simulink model "flyback_switching"  (R2019b)
settings: Solver=FixedStepDiscrete  StartTime=0.0  StopTime=1/60  FixedStep=Ts/1000  MaxStep=1e-4  RelTol=1e-3
values from neighbouring files (symbols this model uses):
  n1 = 2    [final_params.m]
  np = 7    [final_params.m]
  Ts = 1/fsw    (= 1e-05)    [final_params.m]
undefined symbols (not defined in the file or in its folder): C, Cf, duty, fL, Lf, Lm, Vgrms
libraries: powerlib x19, powerlib_meascontrol x1
settings Model: Creator=jvr2131  LastModifiedBy=john
settings DataIOCC: ReturnWorkspaceOutputs=off
settings DebuggingCC: ArithmeticOperatorsInVariantConditions=warning
settings SFSimCC: SimUseLocalCustomCode=off  CustomCodeUndefinedFunction=UseInterfaceOnly
settings RTWCC: RTWUseLocalCustomCode=off

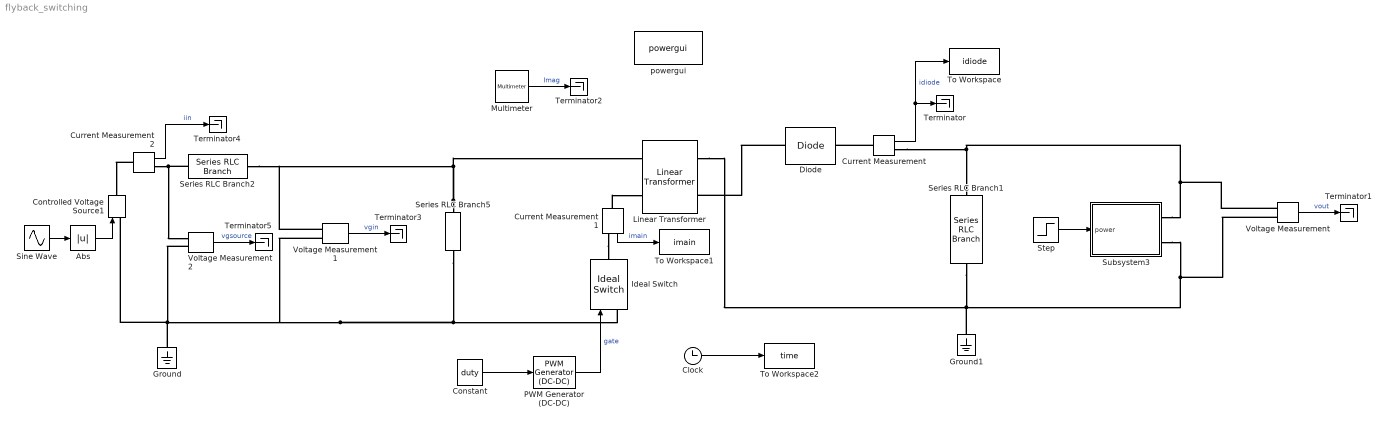
== system flyback_switching ==
  Abs : Abs
  Clock : Clock
  Constant : Constant  Value=duty
  Controlled Voltage Source1 : powerlib/Electrical Sources/Controlled Voltage Source  Initialize=on  Source_Type=AC  Amplitude=0  Phase=0  Frequency=0  Measurements=None
      settings: SourceProductName=Simscape Electrical
  Current Measurement : powerlib/Measurements/Current Measurement  PhasorSimulation=off  OutputType=Complex  PSBequivalent=0
      settings: SourceProductName=Simscape Electrical
  Current Measurement1 : powerlib/Measurements/Current Measurement  PhasorSimulation=off  OutputType=Complex  PSBequivalent=0
      settings: SourceProductName=Simscape Electrical
  Current Measurement2 : powerlib/Measurements/Current Measurement  PhasorSimulation=off  OutputType=Complex  PSBequivalent=0
      settings: SourceProductName=Simscape Electrical
  Diode : powerlib/Power Electronics/Diode  Ron=0.001  Lon=0  Vf=0  IC=0  UseSnubber=0  Rs=500  Cs=0  Measurements=off
      settings: SourceProductName=Simscape Electrical
  Ground : powerlib/Elements/Ground  LConnTagsString=a
      settings: SourceProductName=Simscape Electrical
  Ground1 : powerlib/Elements/Ground  LConnTagsString=a
      settings: SourceProductName=Simscape Electrical
  Ideal Switch : powerlib/Power Electronics/Ideal Switch  Ron=0.001  Lon=0  IC=0  Rs=1e5  Cs=inf  Measurements=off
      settings: SourceProductName=Simscape Electrical
  Linear Transformer : powerlib/Elements/Linear Transformer  UNITS=SI  NominalPower=[ 250e6 60 ]  winding1=[7.35e+05 0 0]  winding2=[(n1/np)*7.35e+05 0 0]  ThreeWindings=off  winding3=[3.15e+05 0.7938 0.084225]  RmLm=[1.0805e+06 Lm]  Measurements=Magnetization current  DataType=on
      settings: SourceProductName=Simscape Electrical
  Multimeter : powerlib/Measurements/Multimeter  PhasorSimulation=off  OutputType=Complex  sel=2  L=3  Gain=1  yselected={'Imag: Linear Transformer'};  PSBOutputType=1  PSBequivalent=0  AxesSetting=[0,0.1,-100,100]  Display=0  SavedBlockNames=-11
      settings: SourceProductName=Simscape Electrical
  PWM Generator (DC-DC) : powerlib_meascontrol/Pulse & Signal Generators/PWM Generator (DC-DC)  Fsw=fs  Ts=0
      settings: SourceProductName=Simscape Electrical
  Series RLC Branch1 : powerlib/Elements/Series RLC Branch  LConnTagsString=__new0  RConnTagsString=__new0  BranchType=C  Resistance=1  Inductance=1e-3  SetiL0=off  InitialCurrent=0  Capacitance=0.1  Setx0=on  InitialVoltage=V  Measurements=None
      settings: SourceProductName=Simscape Electrical
  Series RLC Branch2 : powerlib/Elements/Series RLC Branch  LConnTagsString=__new0  RConnTagsString=__new0  BranchType=L  Resistance=1  Inductance=Lf  SetiL0=off  InitialCurrent=0  Capacitance=C  Setx0=on  InitialVoltage=V  Measurements=None
      settings: SourceProductName=Simscape Electrical
  Series RLC Branch5 : powerlib/Elements/Series RLC Branch  LConnTagsString=__new0  RConnTagsString=__new0  BranchType=C  Resistance=1  Inductance=1e-3  SetiL0=off  InitialCurrent=0  Capacitance=Cf  Setx0=off  InitialVoltage=V  Measurements=None
      settings: SourceProductName=Simscape Electrical
  Sine Wave : Sin  Amplitude=Vgrms*sqrt(2)  Frequency=2*pi*fL  SampleTime=0
  Step : Step  Time=0  Before=power  After=power  SampleTime=0
  Subsystem3 : Subsystem
  Terminator{,1..5} (6 alike) : Terminator
  To Workspace : ToWorkspace  VariableName=idiode  SampleTime=-1
  To Workspace1 : ToWorkspace  VariableName=imain  SampleTime=-1
  To Workspace2 : ToWorkspace  VariableName=time  SampleTime=-1
  Voltage Measurement : powerlib/Measurements/Voltage Measurement  PhasorSimulation=off  OutputType=Complex  PSBequivalent=0
      settings: SourceProductName=Simscape Electrical
  Voltage Measurement1 : powerlib/Measurements/Voltage Measurement  PhasorSimulation=off  OutputType=Complex  PSBequivalent=0
      settings: SourceProductName=Simscape Electrical
  Voltage Measurement2 : powerlib/Measurements/Voltage Measurement  PhasorSimulation=off  OutputType=Complex  PSBequivalent=0
      settings: SourceProductName=Simscape Electrical
  powergui : powerlib/powergui  Priority=1  SimulationMode=Discrete  SampleTime=Ts/1000  frequency=60  Iterations=50  frequencyindice=0  Pbase=100e6  ErrMax=1e-4  UnitsV=kV  UnitsW=MW  buscounter=0  FunctionMessages=off  echomessages=off  EnableUseOfTLC=off  CurrentSourceSwitches=off  DisableSnubberDevices=off  DisableRonSwitches=off  DisableVfSwitches=off  DisplayEquations=off  AutomaticDiscreteSolvers=off  SolverType=Tustin/Backward Euler (TBE)  Interpol=off  ExternalGateDelay=off  methode=off  Ts=100  x0status=blocks  SPID=on  SwTol=0  HookPort=off  NonlinearTolerance=1e-4  nMaxIteration=100  ContinueOnMaxIteration=off  RestoreLinks=warning  ResistiveCurrentMeasurement=off  Frange=[0:2:500]  Ylog=off  Xlog=on  ShowGrid=off  save=off  variable=ZData  structure=0  ZoomFFT=off  StartTime=0.0  cycles=1  DisplayStyle=1  fundamental=60  FreqAxis=off  MaxFrequency=1000  frequencyindicesteady=1  RmsSteady=1  display=off
      settings: SourceProductName=Simscape Electrical
  wires:
  Current Measurement/1 -> To Workspace/1, Terminator/1  "idiode"
  Voltage Measurement/1 -> Terminator1/1  "vout"
  PWM Generator (DC-DC)/1 -> Ideal Switch/1  "gate"
  Constant/1 -> PWM Generator (DC-DC)/1
  Multimeter/1 -> Terminator2/1  "Imag"
  Step/1 -> Subsystem3/1(power)
  Voltage Measurement1/1 -> Terminator3/1  "vgin"
  Current Measurement1/1 -> To Workspace1/1  "imain"
  Sine Wave/1 -> Abs/1
  Abs/1 -> Controlled Voltage Source1/1
  Clock/1 -> To Workspace2/1
  Current Measurement2/1 -> Terminator4/1  "iin"
  Voltage Measurement2/1 -> Terminator5/1  "vgsource"
  connections:
  Series RLC Branch5/RConn1 -- Ideal Switch/LConn1 -- Voltage Measurement2/LConn2 -- Controlled Voltage Source1/LConn1 -- Ground/LConn1 -- Voltage Measurement1/LConn2
  Diode/LConn1 -- Linear Transformer/RConn2
  Voltage Measurement/LConn1 -- Subsystem3/RConn1 -- Current Measurement/RConn1 -- Series RLC Branch1/LConn1
  Series RLC Branch1/RConn1 -- Ground1/LConn1 -- Linear Transformer/RConn1 -- Subsystem3/RConn2 -- Voltage Measurement/LConn2
  Current Measurement/LConn1 -- Diode/RConn1
  Series RLC Branch5/LConn1 -- Series RLC Branch2/RConn1 -- Voltage Measurement1/LConn1 -- Linear Transformer/LConn1
  Current Measurement1/LConn1 -- Linear Transformer/LConn2
  Current Measurement1/RConn1 -- Ideal Switch/RConn1
  Current Measurement2/LConn1 -- Controlled Voltage Source1/RConn1
  Current Measurement2/RConn1 -- Series RLC Branch2/LConn1 -- Voltage Measurement2/LConn1

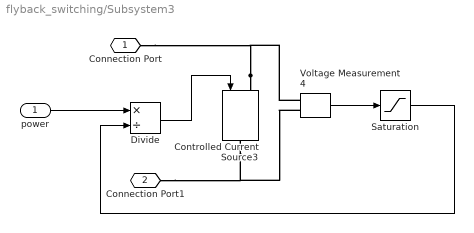
== system flyback_switching/Subsystem3 ==
  power : Inport
  Controlled Current Source3 : powerlib/Electrical Sources/Controlled Current Source  Initialize=on  Source_Type=AC  Amplitude=0  Phase=0  Frequency=0  Measurements=None
      settings: SourceProductName=Simscape Electrical
  Divide : Product  Inputs=*/
  Saturation : Saturate  UpperLimit=inf  LowerLimit=1e-3
  Voltage Measurement4 : powerlib/Measurements/Voltage Measurement  PhasorSimulation=off  OutputType=Complex  PSBequivalent=0
      settings: SourceProductName=Simscape Electrical
  Connection Port : PMIOPort  Side=Right
  Connection Port1 : PMIOPort  Port=2  Side=Right
  wires:
  Saturation/1 -> Divide/2
  power/1 -> Divide/1
  Voltage Measurement4/1 -> Saturation/1
  Divide/1 -> Controlled Current Source3/1
  connections:
  Controlled Current Source3/RConn1 -- Connection Port1/RConn1 -- Voltage Measurement4/LConn2
  Controlled Current Source3/LConn1 -- Connection Port/RConn1 -- Voltage Measurement4/LConn1
